simulink model "soru2"  (R2019b)
settings: Solver=VariableStepAuto  StartTime=0.0  StopTime=50  RelTol=1e-3
libraries: fuzblock x20
settings Model: Creator=Mustafa_Sezer  LastModifiedBy=Mustafa_Sezer
settings SolverCC: AlgebraicLoopSolver=LineSearch

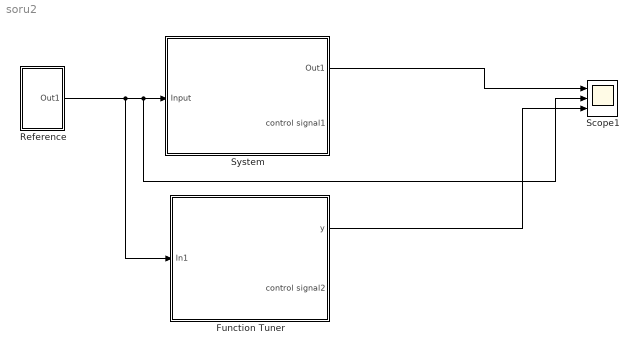
== system soru2 ==
  Function Tuner : Subsystem
  Reference : Subsystem
  Scope1 : Scope  NumInputPorts=3
  System : Subsystem
  wires:
  Function Tuner/1(y) -> Scope1/3
  Reference/1(Out1) -> Function Tuner/1(In1), Scope1/2, System/1(Input)
  System/1(Out1) -> Scope1/1

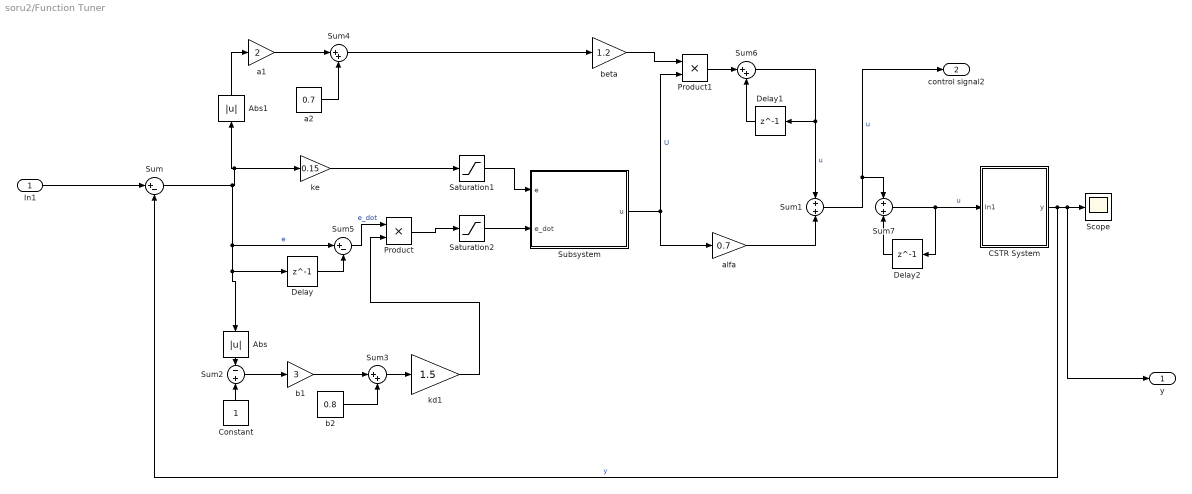
== system soru2/Function Tuner ==
  In1 : Inport
  Abs : Abs
  Abs1 : Abs
  CSTR System : Subsystem
  Constant : Constant  SampleTime=0.01
  Delay : Delay  DelayLength=1  SampleTime=0.1
  Delay1 : Delay  DelayLength=1  SampleTime=0.1
  Delay2 : Delay  DelayLength=1  SampleTime=0.1
  Product : Product
  Product1 : Product
  Saturation1 : Saturate  UpperLimit=1  LowerLimit=-1
  Saturation2 : Saturate  UpperLimit=1  LowerLimit=-1
  Scope : Scope
  Subsystem : Subsystem
  Sum : Sum  Inputs=|+-
  Sum1 : Sum
  Sum2 : Sum  Inputs=-+
  Sum3 : Sum  Inputs=|++
  Sum4 : Sum  Inputs=|++
  Sum5 : Sum  Inputs=|+-
  Sum6 : Sum  Inputs=|++
  Sum7 : Sum
  "a1 " : Gain  Gain=2
  a2 : Constant  Value=0.7  SampleTime=0.1
  "alfa " : Gain  Gain=0.7
  b1 : Gain  Gain=3
  b2 : Constant  Value=0.8  SampleTime=0.1
  beta : Gain  Gain=1.2
  kd1 : Gain  Gain=1.5
  ke : Gain  Gain=0.15
  y : Outport
  control signal2 : Outport  Port=2
  wires:
  "alfa "/1 -> Sum1/2
  ke/1 -> Saturation1/1
  Sum4/1 -> beta/1
  beta/1 -> Product1/1
  kd1/1 -> Product/2
  Product1/1 -> Sum6/1
  Sum3/1 -> kd1/1
  b1/1 -> Sum3/1
  Constant/1 -> Sum2/2
  Sum2/1 -> b1/1
  Abs/1 -> Sum2/1
  "a1 "/1 -> Sum4/1
  Subsystem/1(u) -> "alfa "/1, Product1/2  "U"
  Product/1 -> Saturation2/1
  Abs1/1 -> "a1 "/1
  CSTR System/1(y) -> y/1, Scope/1, Sum/2  "y"
  a2/1 -> Sum4/2
  Sum1/1 -> control signal2/1, Sum7/1  "u"
  b2/1 -> Sum3/2
  In1/1 -> Sum/1
  Saturation1/1 -> Subsystem/1(e)
  Saturation2/1 -> Subsystem/2(e_dot)
  Delay/1 -> Sum5/2
  Sum/1 -> Sum5/1, Abs/1, Delay/1, Abs1/1, ke/1  "e"
  Sum5/1 -> Product/1  "e_dot"
  Sum6/1 -> Delay1/1, Sum1/1  "u"
  Delay1/1 -> Sum6/2
  Delay2/1 -> Sum7/2
  Sum7/1 -> CSTR System/1(In1), Delay2/1  "u"

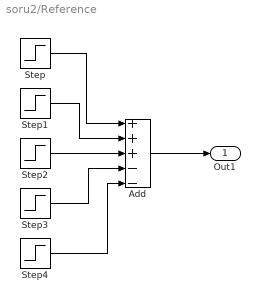
== system soru2/Reference ==
  Add : Sum  Inputs=+++--
  Step : Step  Time=0  After=0.4  SampleTime=0.1
  Step1 : Step  Time=10  After=0.1  SampleTime=0.1
  Step2 : Step  Time=20  After=0.1  SampleTime=0.1
  Step3 : Step  Time=30  After=0.1  SampleTime=0.1
  Step4 : Step  Time=40  After=0.1  SampleTime=0.1
  Out1 : Outport
  wires:
  Step1/1 -> Add/2
  Step/1 -> Add/1
  Add/1 -> Out1/1
  Step3/1 -> Add/4
  Step4/1 -> Add/5
  Step2/1 -> Add/3

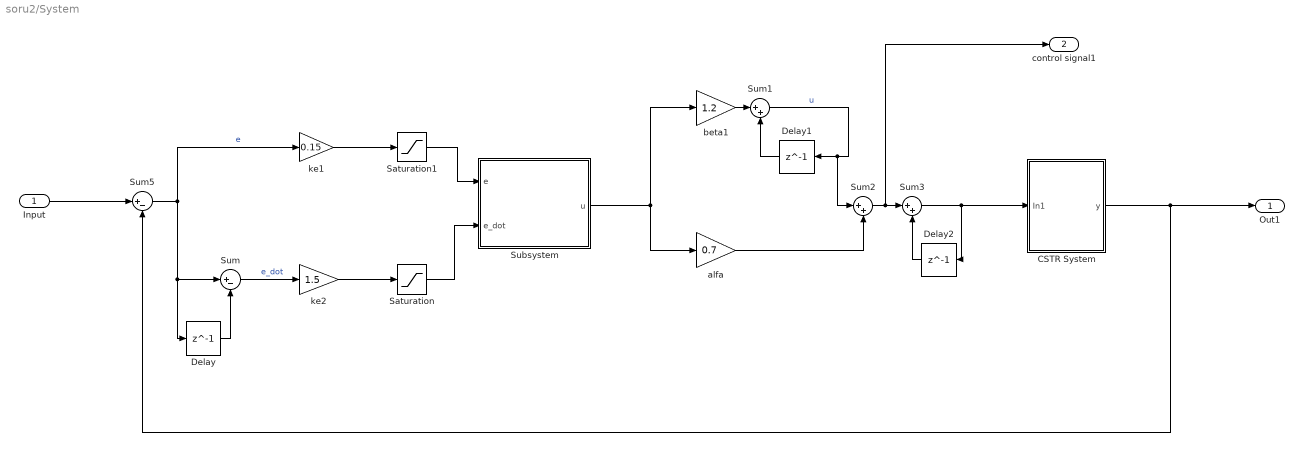
== system soru2/System ==
  Input : Inport
  CSTR System : Subsystem
  Delay : Delay  DelayLength=1  SampleTime=0.1
  Delay1 : Delay  DelayLength=1  SampleTime=0.1
  Delay2 : Delay  DelayLength=1  SampleTime=0.1
  Saturation : Saturate  UpperLimit=1  LowerLimit=-1
  Saturation1 : Saturate  UpperLimit=1  LowerLimit=-1
  Subsystem : Subsystem
  Sum : Sum  Inputs=|+-
  Sum1 : Sum  Inputs=|++
  Sum2 : Sum  Inputs=|++
  Sum3 : Sum  Inputs=|++
  Sum5 : Sum  Inputs=|+-
  alfa : Gain  Gain=0.7
  beta1 : Gain  Gain=1.2
  ke1 : Gain  Gain=0.15
  ke2 : Gain  Gain=1.5
  Out1 : Outport
  control signal1 : Outport  Port=2
  wires:
  beta1/1 -> Sum1/1
  Sum/1 -> ke2/1  "e_dot"
  Input/1 -> Sum5/1
  Sum5/1 -> Delay/1, Sum/1, ke1/1  "e"
  Sum1/1 -> Sum2/1, Delay1/1  "u"
  Subsystem/1(u) -> beta1/1, alfa/1
  ke1/1 -> Saturation1/1
  ke2/1 -> Saturation/1
  Delay/1 -> Sum/2
  Delay1/1 -> Sum1/2
  Saturation/1 -> Subsystem/2(e_dot)
  Sum2/1 -> control signal1/1, Sum3/1
  alfa/1 -> Sum2/2
  Saturation1/1 -> Subsystem/1(e)
  Sum3/1 -> Delay2/1, CSTR System/1(In1)
  Delay2/1 -> Sum3/2
  CSTR System/1(y) -> Sum5/2, Out1/1

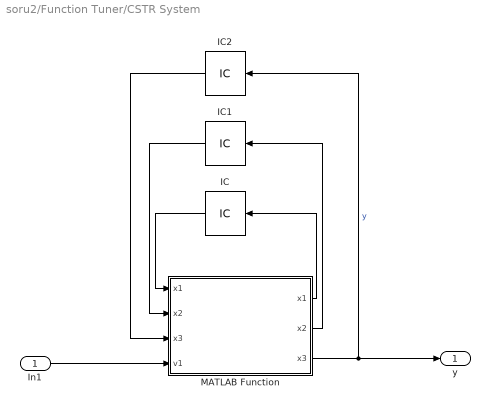
== system soru2/Function Tuner/CSTR System ==
  In1 : Inport
  IC : InitialCondition  Value=0.31
  IC1 : InitialCondition  Value=0.71
  IC2 : InitialCondition  Value=0.5
  MATLAB Function : MATLAB Function  TreatAsAtomicUnit=on
  y : Outport
  wires:
  IC1/1 -> MATLAB Function/2("x2 ")
  MATLAB Function/2(x2) -> IC1/1
  IC/1 -> MATLAB Function/1("x1 ")
  In1/1 -> MATLAB Function/4(v1)
  MATLAB Function/1(x1) -> IC/1
  IC2/1 -> MATLAB Function/3("x3 ")
  MATLAB Function/3(x3) -> y/1, IC2/1  "y"

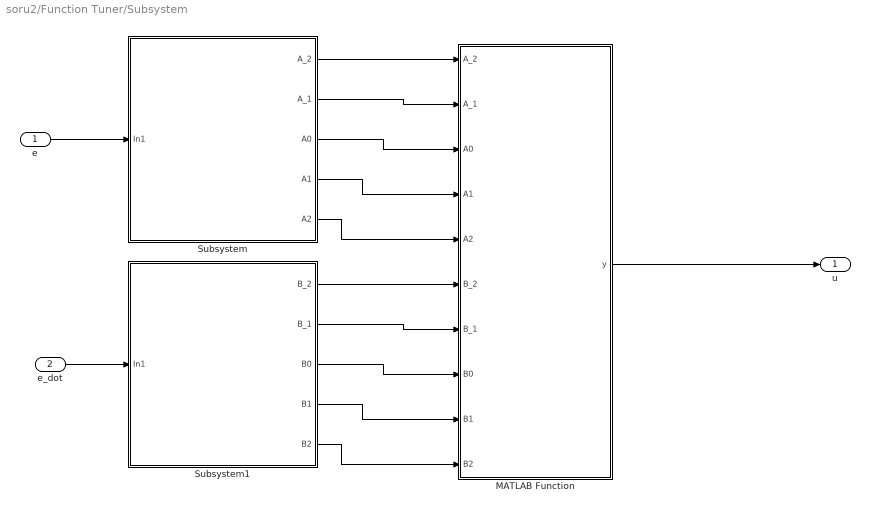
== system soru2/Function Tuner/Subsystem ==
  e : Inport
  e_dot : Inport  Port=2
  MATLAB Function : MATLAB Function  TreatAsAtomicUnit=on
  Subsystem : Subsystem
  Subsystem1 : Subsystem
  u : Outport
  wires:
  MATLAB Function/1(y) -> u/1
  Subsystem/5(A2) -> MATLAB Function/5(A2)
  Subsystem/4(A1) -> MATLAB Function/4(A1)
  Subsystem/3(A0) -> MATLAB Function/3(A0)
  Subsystem/2(A_1) -> MATLAB Function/2(A_1)
  Subsystem/1(A_2) -> MATLAB Function/1(A_2)
  Subsystem1/1(B_2) -> MATLAB Function/6(B_2)
  Subsystem1/2(B_1) -> MATLAB Function/7(B_1)
  Subsystem1/3(B0) -> MATLAB Function/8(B0)
  Subsystem1/4(B1) -> MATLAB Function/9(B1)
  Subsystem1/5(B2) -> MATLAB Function/10(B2)
  e/1 -> Subsystem/1(In1)
  e_dot/1 -> Subsystem1/1(In1)

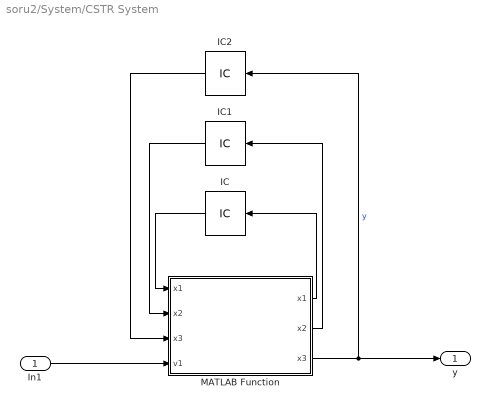
== system soru2/System/CSTR System ==
  In1 : Inport
  IC : InitialCondition  Value=0.31
  IC1 : InitialCondition  Value=0.71
  IC2 : InitialCondition  Value=0.5
  MATLAB Function : MATLAB Function  TreatAsAtomicUnit=on
  y : Outport
  wires:
  IC1/1 -> MATLAB Function/2("x2 ")
  MATLAB Function/2(x2) -> IC1/1
  IC/1 -> MATLAB Function/1("x1 ")
  In1/1 -> MATLAB Function/4(v1)
  MATLAB Function/1(x1) -> IC/1
  IC2/1 -> MATLAB Function/3("x3 ")
  MATLAB Function/3(x3) -> y/1, IC2/1  "y"

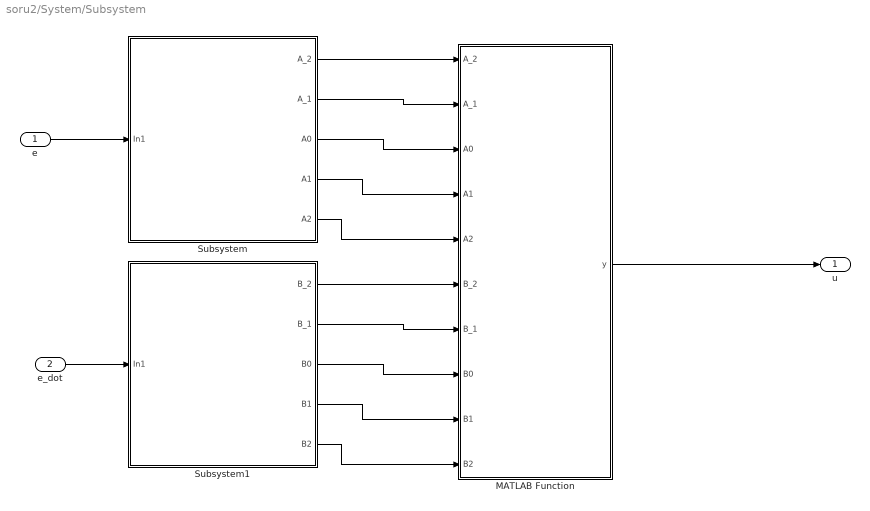
== system soru2/System/Subsystem ==
  e : Inport
  e_dot : Inport  Port=2
  MATLAB Function : MATLAB Function  TreatAsAtomicUnit=on
  Subsystem : Subsystem
  Subsystem1 : Subsystem
  u : Outport
  wires:
  MATLAB Function/1(y) -> u/1
  Subsystem/5(A2) -> MATLAB Function/5(A2)
  Subsystem/4(A1) -> MATLAB Function/4(A1)
  Subsystem/3(A0) -> MATLAB Function/3(A0)
  Subsystem/2(A_1) -> MATLAB Function/2(A_1)
  Subsystem/1(A_2) -> MATLAB Function/1(A_2)
  Subsystem1/1(B_2) -> MATLAB Function/6(B_2)
  Subsystem1/2(B_1) -> MATLAB Function/7(B_1)
  Subsystem1/3(B0) -> MATLAB Function/8(B0)
  Subsystem1/4(B1) -> MATLAB Function/9(B1)
  Subsystem1/5(B2) -> MATLAB Function/10(B2)
  e/1 -> Subsystem/1(In1)
  e_dot/1 -> Subsystem1/1(In1)

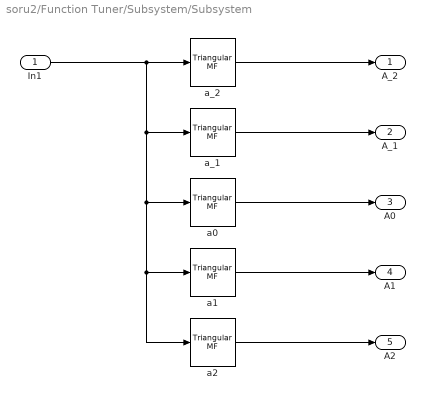
== system soru2/Function Tuner/Subsystem/Subsystem ==
  In1 : Inport
  a0 : fuzblock/Membership  Functions/Triangular MF  a=-0.4  b=0  c=0.4
      settings: SourceProductName=Fuzzy Logic Toolbox  SourceProductBaseCode=FL
  a1 : fuzblock/Membership  Functions/Triangular MF  a=0  b=0.4  c=1
      settings: SourceProductName=Fuzzy Logic Toolbox  SourceProductBaseCode=FL
  a2 : fuzblock/Membership  Functions/Triangular MF  a=0.4  b=1  c=1
      settings: SourceProductName=Fuzzy Logic Toolbox  SourceProductBaseCode=FL
  a_1 : fuzblock/Membership  Functions/Triangular MF  a=-1  b=-0.4  c=0
      settings: SourceProductName=Fuzzy Logic Toolbox  SourceProductBaseCode=FL
  a_2 : fuzblock/Membership  Functions/Triangular MF  a=-1  b=-1  c=-0.4
      settings: SourceProductName=Fuzzy Logic Toolbox  SourceProductBaseCode=FL
  A_2 : Outport
  A_1 : Outport  Port=2
  A0 : Outport  Port=3
  A1 : Outport  Port=4
  A2 : Outport  Port=5
  wires:
  a_2/1 -> A_2/1
  a1/1 -> A1/1
  a2/1 -> A2/1
  a_1/1 -> A_1/1
  a0/1 -> A0/1
  In1/1 -> a2/1, a1/1, a0/1, a_1/1, a_2/1

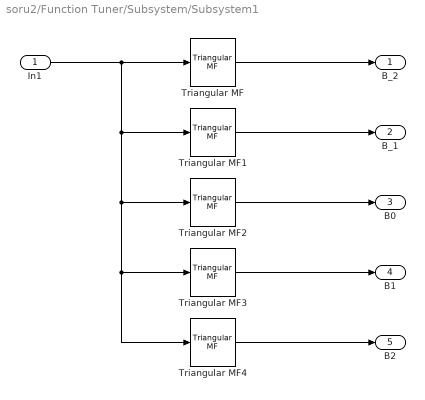
== system soru2/Function Tuner/Subsystem/Subsystem1 ==
  In1 : Inport
  Triangular MF : fuzblock/Membership  Functions/Triangular MF  a=-1  b=-1  c=-0.4
      settings: SourceProductName=Fuzzy Logic Toolbox  SourceProductBaseCode=FL
  Triangular MF1 : fuzblock/Membership  Functions/Triangular MF  a=-1  b=-0.4  c=0
      settings: SourceProductName=Fuzzy Logic Toolbox  SourceProductBaseCode=FL
  Triangular MF2 : fuzblock/Membership  Functions/Triangular MF  a=-0.4  b=0  c=0.4
      settings: SourceProductName=Fuzzy Logic Toolbox  SourceProductBaseCode=FL
  Triangular MF3 : fuzblock/Membership  Functions/Triangular MF  a=0  b=0.4  c=1
      settings: SourceProductName=Fuzzy Logic Toolbox  SourceProductBaseCode=FL
  Triangular MF4 : fuzblock/Membership  Functions/Triangular MF  a=0.4  b=1  c=1
      settings: SourceProductName=Fuzzy Logic Toolbox  SourceProductBaseCode=FL
  B_2 : Outport
  B_1 : Outport  Port=2
  B0 : Outport  Port=3
  B1 : Outport  Port=4
  B2 : Outport  Port=5
  wires:
  In1/1 -> Triangular MF4/1, Triangular MF3/1, Triangular MF2/1, Triangular MF1/1, Triangular MF/1
  Triangular MF/1 -> B_2/1
  Triangular MF4/1 -> B2/1
  Triangular MF2/1 -> B0/1
  Triangular MF1/1 -> B_1/1
  Triangular MF3/1 -> B1/1

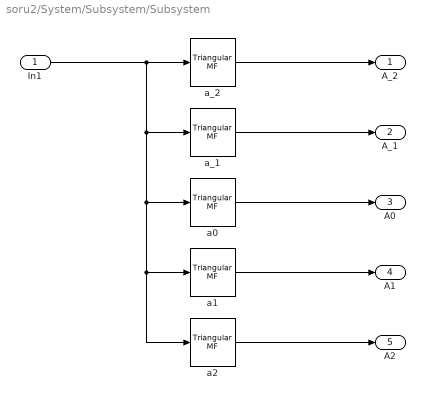
== system soru2/System/Subsystem/Subsystem ==
  In1 : Inport
  a0 : fuzblock/Membership  Functions/Triangular MF  a=-0.4  b=0  c=0.4
      settings: SourceProductName=Fuzzy Logic Toolbox  SourceProductBaseCode=FL
  a1 : fuzblock/Membership  Functions/Triangular MF  a=0  b=0.4  c=1
      settings: SourceProductName=Fuzzy Logic Toolbox  SourceProductBaseCode=FL
  a2 : fuzblock/Membership  Functions/Triangular MF  a=0.4  b=1  c=1
      settings: SourceProductName=Fuzzy Logic Toolbox  SourceProductBaseCode=FL
  a_1 : fuzblock/Membership  Functions/Triangular MF  a=-1  b=-0.4  c=0
      settings: SourceProductName=Fuzzy Logic Toolbox  SourceProductBaseCode=FL
  a_2 : fuzblock/Membership  Functions/Triangular MF  a=-1  b=-1  c=-0.4
      settings: SourceProductName=Fuzzy Logic Toolbox  SourceProductBaseCode=FL
  A_2 : Outport
  A_1 : Outport  Port=2
  A0 : Outport  Port=3
  A1 : Outport  Port=4
  A2 : Outport  Port=5
  wires:
  a_2/1 -> A_2/1
  a1/1 -> A1/1
  a2/1 -> A2/1
  a_1/1 -> A_1/1
  a0/1 -> A0/1
  In1/1 -> a2/1, a1/1, a0/1, a_1/1, a_2/1

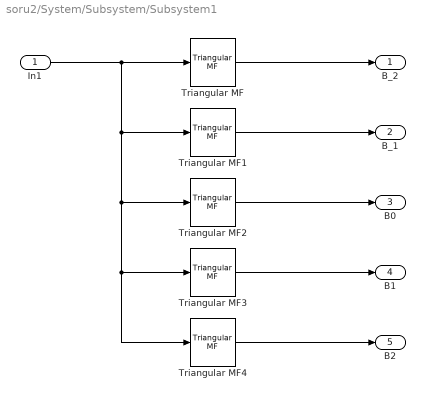
== system soru2/System/Subsystem/Subsystem1 ==
  In1 : Inport
  Triangular MF : fuzblock/Membership  Functions/Triangular MF  a=-1  b=-1  c=-0.4
      settings: SourceProductName=Fuzzy Logic Toolbox  SourceProductBaseCode=FL
  Triangular MF1 : fuzblock/Membership  Functions/Triangular MF  a=-1  b=-0.4  c=0
      settings: SourceProductName=Fuzzy Logic Toolbox  SourceProductBaseCode=FL
  Triangular MF2 : fuzblock/Membership  Functions/Triangular MF  a=-0.4  b=0  c=0.4
      settings: SourceProductName=Fuzzy Logic Toolbox  SourceProductBaseCode=FL
  Triangular MF3 : fuzblock/Membership  Functions/Triangular MF  a=0  b=0.4  c=1
      settings: SourceProductName=Fuzzy Logic Toolbox  SourceProductBaseCode=FL
  Triangular MF4 : fuzblock/Membership  Functions/Triangular MF  a=0.4  b=1  c=1
      settings: SourceProductName=Fuzzy Logic Toolbox  SourceProductBaseCode=FL
  B_2 : Outport
  B_1 : Outport  Port=2
  B0 : Outport  Port=3
  B1 : Outport  Port=4
  B2 : Outport  Port=5
  wires:
  In1/1 -> Triangular MF4/1, Triangular MF3/1, Triangular MF2/1, Triangular MF1/1, Triangular MF/1
  Triangular MF/1 -> B_2/1
  Triangular MF4/1 -> B2/1
  Triangular MF2/1 -> B0/1
  Triangular MF1/1 -> B_1/1
  Triangular MF3/1 -> B1/1

== matlab function soru2/System/Subsystem/MATLAB Function ==
  data: A_2 input; y output; A_1 input; A0 input; A1 input; A2 input; B_2 input; B_1 input; B0 input; B1 input; B2 input
function y = fcn(A_2, A_1, A0, A1, A2, B_2, B_1, B0, B1, B2)
u_2_2 = -1;
u_2_1 = -0.7;
u_20 = -0.5;
u_21 = -0.3;
u_22 = 0;

u_1_2 = -0.7;
u_1_1 = -0.4;
u_10 = -0.2;
u_11 = 0;
u_12 = 0.3;

u0_2 = -0.5;
u0_1 = -0.2;
u00 = 0;
u01 = 0.2;
u02 = 0.5;

u1_2 = -0.3;
u1_1 = 0;
u10 = 0.2;
u11 = 0.4;
u12 = 0.7;

u2_2 = 0;
u2_1 = 0.3;
u20 = 0.5;
u21 = 0.7;
u22 = 1;

if ((A0==0) && (A1==0) && (A2==0)) % A_1 ve A_2
    
    if((B0==0) && (B1==0) && (B2==0) && (B_1~= 0) && (B_2~= 0))
        y = A_2*B_2*u_2_2 + A_2*B_1*u_2_1 + A_1*B_1*u_1_1 + A_1*B_2*u_1_2;
    
    elseif((B_2==0) && (B1==0) && (B2==0) && (B_1~= 0) && (B0~= 0))
        y = A_2*B_1*u_2_1 + A_2*B0*u_20 + A_1*B_1*u_1_1 + A_1*B0*u_10;
    
    elseif((B_2==0) && (B_1==0) && (B2==0) && (B0~= 0) && (B1~= 0))
        y = A_2*B0*u_20 + A_2*B1*u_21 + A_1*B0*u_10 + A_1*B1*u_11;
    
    elseif((B0==0) && (B_1==0) && (B_2==0) && (B1~= 0) && (B2~= 0))
        y = A_2*B1*u_21 + A_2*B2*u_22 + A_1*B1*u_11 + A_1*B2*u_12;
    
    elseif((B_1==0) && (B0==0) && (B1==0) && (B2==0))
        y = A_2*B_2*u_2_2 + A_1*B_2*u_1_2;
    
    elseif((B_2==0) && (B0==0) && (B1==0) && (B2==0))
        y = A_2*B_1*u_2_1 + A_1*B_1*u_1_1;
    
    elseif((B_2==0) && (B_1==0) && (B1==0) && (B2==0))
        y = A_2*B0*u_20 + A_1*B0*u_10;
    
    elseif((B_2==0) && (B_1==0) && (B0==0) && (B2==0))
        y = A_2*B1*u_21 + A_1*B1*u_11;
    
    elseif((B_2==0) && (B_1==0) && (B0==0) && (B1==0))
        y = A_2*B2*u_22 + A_1*B2*u_12;
    
    else
        y=0.5;
    end
    
elseif ((A_2==0) && (A1==0) && (A2==0)) % A_1 ve A0
    
    if((B0==0) && (B1==0) && (B2==0) && (B_1~= 0) && (B_2~= 0))
        y = A0*B_2*u0_2 + A0*B_1*u0_1 + A_1*B_1*u_1_1 + A_1*B_2*u_1_2;
    
    elseif((B_2==0) && (B1==0) && (B2==0) && (B_1~= 0) && (B0~= 0))
        y = A0*B_1*u0_1 + A0*B0*u00 + A_1*B_1*u_1_1 + A_1*B0*u_10;
    
    elseif((B_2==0) && (B_1==0) && (B2==0) && (B0~= 0) && (B1~= 0))
        y = A0*B0*u00 + A0*B1*u01 + A_1*B0*u_10 + A_1*B1*u_11;
    
    elseif((B0==0) && (B_1==0) && (B_2==0) && (B1~= 0) && (B2~= 0))
        y = A0*B1*u01 + A0*B2*u02 + A_1*B1*u_11 + A_1*B2*u_12;
    
    elseif((B_1==0) && (B0==0) && (B1==0) && (B2==0))
        y = A0*B_2*u0_2 + A_1*B_2*u_1_2;
    
    elseif((B_2==0) && (B0==0) && (B1==0) && (B2==0))
        y = A0*B_1*u0_1 + A_1*B_1*u_1_1;
    
    elseif((B_2==0) && (B_1==0) && (B1==0) && (B2==0))
        y = A0*B0*u00 + A_1*B0*u_10;
    
    elseif((B_2==0) && (B_1==0) && (B0==0) && (B2==0))
        y = A0*B1*u01 + A_1*B1*u_11;
    
    elseif((B_2==0) && (B_1==0) && (B0==0) && (B1==0))
        y = A0*B2*u02 + A_1*B2*u_12;
    
    else
        y=0.5;
    end
    
elseif ((A_2==0) && (A_1==0) && (A2==0)) % A1 ve A0
    
    if((B0==0) && (B1==0) && (B2==0) && (B_1~= 0) && (B_2~= 0))
        y = A0*B_2*u0_2 + A0*B_1*u0_1 + A1*B_1*u1_1 + A1*B_2*u1_2;
    
    elseif((B_2==0) && (B1==0) && (B2==0) && (B_1~= 0) && (B0~= 0))
        y = A0*B_1*u0_1 + A0*B0*u00 + A1*B_1*u1_1 + A1*B0*u10;
    
    elseif((B_2==0) && (B_1==0) && (B2==0) && (B0~= 0) && (B1~= 0))
        y = A0*B0*u00 + A0*B1*u01 + A1*B0*u10 + A1*B1*u11;
    
    elseif((B0==0) && (B_1==0) && (B_2==0) && (B1~= 0) && (B2~= 0))
        y = A0*B1*u01 + A0*B2*u02 + A1*B1*u11 + A1*B2*u12;
    
    elseif((B_1==0) && (B0==0) && (B1==0) && (B2==0))
        y = A0*B_2*u0_2 + A1*B_2*u1_2;
    
    elseif((B_2==0) && (B0==0) && (B1==0) && (B2==0))
        y = A0*B_1*u0_1 + A1*B_1*u1_1;
    
    elseif((B_2==0) && (B_1==0) && (B1==0) && (B2==0))
        y = A0*B0*u00 + A1*B0*u10;
    
    elseif((B_2==0) && (B_1==0) && (B0==0) && (B2==0))
        y = A0*B1*u01 + A1*B1*u11;
    
    elseif((B_2==0) && (B_1==0) && (B0==0) && (B1==0))
        y = A0*B2*u02 + A1*B2*u12;
    
    else
        y=0.5;
    end
    
elseif ((A_2==0) && (A_1==0) && (A0==0)) % A1 ve A2
    
    if((B0==0) && (B1==0) && (B2==0) && (B_1~= 0) && (B_2~= 0))
        y = A2*B_2*u2_2 + A2*B_1*u2_1 + A1*B_1*u1_1 + A1*B_2*u1_2;
    
    elseif((B_2==0) && (B1==0) && (B2==0) && (B_1~= 0) && (B0~= 0))
        y = A2*B_1*u2_1 + A2*B0*u20 + A1*B_1*u1_1 + A1*B0*u10;
    
    elseif((B_2==0) && (B_1==0) && (B2==0) && (B0~= 0) && (B1~= 0))
        y = A2*B0*u20 + A2*B1*u21 + A1*B0*u10 + A1*B1*u11;
    
    elseif((B0==0) && (B_1==0) && (B_2==0) && (B1~= 0) && (B2~= 0))
        y = A2*B1*u21 + A2*B2*u22 + A1*B1*u11 + A1*B2*u12;
    
    elseif((B_1==0) && (B0==0) && (B1==0) && (B2==0))
        y = A2*B_2*u2_2 + A1*B_2*u1_2;
    
    elseif((B_2==0) && (B0==0) && (B1==0) && (B2==0))
        y = A2*B_1*u2_1 + A1*B_1*u1_1;
    
    elseif((B_2==0) && (B_1==0) && (B1==0) && (B2==0))
        y = A2*B0*u20 + A1*B0*u10;
    
    elseif((B_2==0) && (B_1==0) && (B0==0) && (B2==0))
        y = A2*B1*u21 + A1*B1*u11;
    
    elseif((B_2==0) && (B_1==0) && (B0==0) && (B1==0))
        y = A2*B2*u22 + A1*B2*u12;
    
    else
        y=0.5;
    end
else
    y=0.5;
end

== matlab function soru2/System/CSTR System/MATLAB Function ==
  data: x1 input; x1 output; x2 input; x3 input; v1 input; x2 output; x3 output
% Runge Kutta method for CSTR 
% Da1, Da2, Da3, d2 are CSTR parameters
% v1 is control input.
% h is the sampling time.
% x1, x2, x3 are the states of the system.

function  [x1,x2,x3]=CSTR_runga_kutta_new(x1,x2,x3,v1)
Da1 = 3; Da2 = 0.5; Da3 = 1; d2 = 1; h = 0.1;

k1x1=1-x1-Da1*x1+Da2*x2*x2;
k1x2=-x2+Da1*x1-Da2*x2*x2-Da3*d2*x2*x2+v1;
k1x3=-x3+Da3*d2*x2*x2;



k2x1=1-(x1+h*k1x1/2)-Da1*(x1+h*k1x1/2)+Da2*(x2+h*k1x2/2)*(x2+h*k1x2/2);
k2x2=-(x2+h*k1x2/2)+Da1*(x1+h*k1x1/2)-Da2*(x2+h*k1x2/2)*(x2+h*k1x2/2)-Da3*d2*(x2+h*k1x2/2)*(x2+h*k1x2/2)+v1;
k2x3=-(x3+h*k1x3/2 )+Da3*d2*(x2+h*k1x2/2)*(x2+h*k1x2/2);


k3x1=1-(x1+h*k2x1/2)-Da1*(x1+h*k2x1/2)+Da2*(x2+h*k2x2/2)*(x2+h*k2x2/2);
k3x2=-(x2+h*k2x2/2)+Da1*(x1+h*k2x1/2)-Da2*(x2+h*k2x2/2)*(x2+h*k2x2/2)-Da3*d2*(x2+h*k2x2/2)*(x2+h*k2x2/2)+v1;
k3x3=-(x3+h*k2x3/2)+Da3*d2*(x2+h*k2x2/2)*(x2+h*k2x2/2);



k4x1=1-(x1+h*k3x1)-Da1*(x1+h*k3x1)+Da2*(x2+h*k3x2)*(x2+h*k3x2);
k4x2=-(x2+h*k3x2)+Da1*(x1+h*k3x1)-Da2*(x2+h*k3x2)*(x2+h*k3x2)-Da3*d2*(x2+h*k3x2)*(x2+h*k3x2)+v1;
k4x3=-(x3+h*k3x3)+Da3*d2*(x2+h*k3x2)*(x2+h*k3x2);



x1=x1+(h/6)*(k1x1+2*k2x1+2*k3x1+k4x1);
x2=x2+(h/6)*(k1x2+2*k2x2+2*k3x2+k4x2);
x3=x3+(h/6)*(k1x3+2*k2x3+2*k3x3+k4x3);

== matlab function soru2/Function Tuner/Subsystem/MATLAB Function ==
  data: A_2 input; y output; A_1 input; A0 input; A1 input; A2 input; B_2 input; B_1 input; B0 input; B1 input; B2 input
function y = fcn(A_2, A_1, A0, A1, A2, B_2, B_1, B0, B1, B2)
u_2_2 = -1;
u_2_1 = -0.7;
u_20 = -0.5;
u_21 = -0.3;
u_22 = 0;

u_1_2 = -0.7;
u_1_1 = -0.4;
u_10 = -0.2;
u_11 = 0;
u_12 = 0.3;

u0_2 = -0.5;
u0_1 = -0.2;
u00 = 0;
u01 = 0.2;
u02 = 0.5;

u1_2 = -0.3;
u1_1 = 0;
u10 = 0.2;
u11 = 0.4;
u12 = 0.7;

u2_2 = 0;
u2_1 = 0.3;
u20 = 0.5;
u21 = 0.7;
u22 = 1;

if ((A0==0) && (A1==0) && (A2==0)) % A_1 ve A_2
    
    if((B0==0) && (B1==0) && (B2==0) && (B_1~= 0) && (B_2~= 0))
        y = A_2*B_2*u_2_2 + A_2*B_1*u_2_1 + A_1*B_1*u_1_1 + A_1*B_2*u_1_2;
    
    elseif((B_2==0) && (B1==0) && (B2==0) && (B_1~= 0) && (B0~= 0))
        y = A_2*B_1*u_2_1 + A_2*B0*u_20 + A_1*B_1*u_1_1 + A_1*B0*u_10;
    
    elseif((B_2==0) && (B_1==0) && (B2==0) && (B0~= 0) && (B1~= 0))
        y = A_2*B0*u_20 + A_2*B1*u_21 + A_1*B0*u_10 + A_1*B1*u_11;
    
    elseif((B0==0) && (B_1==0) && (B_2==0) && (B1~= 0) && (B2~= 0))
        y = A_2*B1*u_21 + A_2*B2*u_22 + A_1*B1*u_11 + A_1*B2*u_12;
    
    elseif((B_1==0) && (B0==0) && (B1==0) && (B2==0))
        y = A_2*B_2*u_2_2 + A_1*B_2*u_1_2;
    
    elseif((B_2==0) && (B0==0) && (B1==0) && (B2==0))
        y = A_2*B_1*u_2_1 + A_1*B_1*u_1_1;
    
    elseif((B_2==0) && (B_1==0) && (B1==0) && (B2==0))
        y = A_2*B0*u_20 + A_1*B0*u_10;
    
    elseif((B_2==0) && (B_1==0) && (B0==0) && (B2==0))
        y = A_2*B1*u_21 + A_1*B1*u_11;
    
    elseif((B_2==0) && (B_1==0) && (B0==0) && (B1==0))
        y = A_2*B2*u_22 + A_1*B2*u_12;
    
    else
        y=0.5;
    end
    
elseif ((A_2==0) && (A1==0) && (A2==0)) % A_1 ve A0
    
    if((B0==0) && (B1==0) && (B2==0) && (B_1~= 0) && (B_2~= 0))
        y = A0*B_2*u0_2 + A0*B_1*u0_1 + A_1*B_1*u_1_1 + A_1*B_2*u_1_2;
    
    elseif((B_2==0) && (B1==0) && (B2==0) && (B_1~= 0) && (B0~= 0))
        y = A0*B_1*u0_1 + A0*B0*u00 + A_1*B_1*u_1_1 + A_1*B0*u_10;
    
    elseif((B_2==0) && (B_1==0) && (B2==0) && (B0~= 0) && (B1~= 0))
        y = A0*B0*u00 + A0*B1*u01 + A_1*B0*u_10 + A_1*B1*u_11;
    
    elseif((B0==0) && (B_1==0) && (B_2==0) && (B1~= 0) && (B2~= 0))
        y = A0*B1*u01 + A0*B2*u02 + A_1*B1*u_11 + A_1*B2*u_12;
    
    elseif((B_1==0) && (B0==0) && (B1==0) && (B2==0))
        y = A0*B_2*u0_2 + A_1*B_2*u_1_2;
    
    elseif((B_2==0) && (B0==0) && (B1==0) && (B2==0))
        y = A0*B_1*u0_1 + A_1*B_1*u_1_1;
    
    elseif((B_2==0) && (B_1==0) && (B1==0) && (B2==0))
        y = A0*B0*u00 + A_1*B0*u_10;
    
    elseif((B_2==0) && (B_1==0) && (B0==0) && (B2==0))
        y = A0*B1*u01 + A_1*B1*u_11;
    
    elseif((B_2==0) && (B_1==0) && (B0==0) && (B1==0))
        y = A0*B2*u02 + A_1*B2*u_12;
    
    else
        y=0.5;
    end
    
elseif ((A_2==0) && (A_1==0) && (A2==0)) % A1 ve A0
    
    if((B0==0) && (B1==0) && (B2==0) && (B_1~= 0) && (B_2~= 0))
        y = A0*B_2*u0_2 + A0*B_1*u0_1 + A1*B_1*u1_1 + A1*B_2*u1_2;
    
    elseif((B_2==0) && (B1==0) && (B2==0) && (B_1~= 0) && (B0~= 0))
        y = A0*B_1*u0_1 + A0*B0*u00 + A1*B_1*u1_1 + A1*B0*u10;
    
    elseif((B_2==0) && (B_1==0) && (B2==0) && (B0~= 0) && (B1~= 0))
        y = A0*B0*u00 + A0*B1*u01 + A1*B0*u10 + A1*B1*u11;
    
    elseif((B0==0) && (B_1==0) && (B_2==0) && (B1~= 0) && (B2~= 0))
        y = A0*B1*u01 + A0*B2*u02 + A1*B1*u11 + A1*B2*u12;
    
    elseif((B_1==0) && (B0==0) && (B1==0) && (B2==0))
        y = A0*B_2*u0_2 + A1*B_2*u1_2;
    
    elseif((B_2==0) && (B0==0) && (B1==0) && (B2==0))
        y = A0*B_1*u0_1 + A1*B_1*u1_1;
    
    elseif((B_2==0) && (B_1==0) && (B1==0) && (B2==0))
        y = A0*B0*u00 + A1*B0*u10;
    
    elseif((B_2==0) && (B_1==0) && (B0==0) && (B2==0))
        y = A0*B1*u01 + A1*B1*u11;
    
    elseif((B_2==0) && (B_1==0) && (B0==0) && (B1==0))
        y = A0*B2*u02 + A1*B2*u12;
    
    else
        y=0.5;
    end
    
elseif ((A_2==0) && (A_1==0) && (A0==0)) % A1 ve A2
    
    if((B0==0) && (B1==0) && (B2==0) && (B_1~= 0) && (B_2~= 0))
        y = A2*B_2*u2_2 + A2*B_1*u2_1 + A1*B_1*u1_1 + A1*B_2*u1_2;
    
    elseif((B_2==0) && (B1==0) && (B2==0) && (B_1~= 0) && (B0~= 0))
        y = A2*B_1*u2_1 + A2*B0*u20 + A1*B_1*u1_1 + A1*B0*u10;
    
    elseif((B_2==0) && (B_1==0) && (B2==0) && (B0~= 0) && (B1~= 0))
        y = A2*B0*u20 + A2*B1*u21 + A1*B0*u10 + A1*B1*u11;
    
    elseif((B0==0) && (B_1==0) && (B_2==0) && (B1~= 0) && (B2~= 0))
        y = A2*B1*u21 + A2*B2*u22 + A1*B1*u11 + A1*B2*u12;
    
    elseif((B_1==0) && (B0==0) && (B1==0) && (B2==0))
        y = A2*B_2*u2_2 + A1*B_2*u1_2;
    
    elseif((B_2==0) && (B0==0) && (B1==0) && (B2==0))
        y = A2*B_1*u2_1 + A1*B_1*u1_1;
    
    elseif((B_2==0) && (B_1==0) && (B1==0) && (B2==0))
        y = A2*B0*u20 + A1*B0*u10;
    
    elseif((B_2==0) && (B_1==0) && (B0==0) && (B2==0))
        y = A2*B1*u21 + A1*B1*u11;
    
    elseif((B_2==0) && (B_1==0) && (B0==0) && (B1==0))
        y = A2*B2*u22 + A1*B2*u12;
    
    else
        y=0.5;
    end
else
    y=0.5;
end

== matlab function soru2/Function Tuner/CSTR System/MATLAB Function ==
  data: x1 input; x1 output; x2 input; x3 input; v1 input; x2 output; x3 output
% Runge Kutta method for CSTR 
% Da1, Da2, Da3, d2 are CSTR parameters
% v1 is control input.
% h is the sampling time.
% x1, x2, x3 are the states of the system.

function  [x1,x2,x3]=CSTR_runga_kutta_new(x1,x2,x3,v1)
Da1 = 3; Da2 = 0.5; Da3 = 1; d2 = 1; h = 0.1;

k1x1=1-x1-Da1*x1+Da2*x2*x2;
k1x2=-x2+Da1*x1-Da2*x2*x2-Da3*d2*x2*x2+v1;
k1x3=-x3+Da3*d2*x2*x2;



k2x1=1-(x1+h*k1x1/2)-Da1*(x1+h*k1x1/2)+Da2*(x2+h*k1x2/2)*(x2+h*k1x2/2);
k2x2=-(x2+h*k1x2/2)+Da1*(x1+h*k1x1/2)-Da2*(x2+h*k1x2/2)*(x2+h*k1x2/2)-Da3*d2*(x2+h*k1x2/2)*(x2+h*k1x2/2)+v1;
k2x3=-(x3+h*k1x3/2 )+Da3*d2*(x2+h*k1x2/2)*(x2+h*k1x2/2);


k3x1=1-(x1+h*k2x1/2)-Da1*(x1+h*k2x1/2)+Da2*(x2+h*k2x2/2)*(x2+h*k2x2/2);
k3x2=-(x2+h*k2x2/2)+Da1*(x1+h*k2x1/2)-Da2*(x2+h*k2x2/2)*(x2+h*k2x2/2)-Da3*d2*(x2+h*k2x2/2)*(x2+h*k2x2/2)+v1;
k3x3=-(x3+h*k2x3/2)+Da3*d2*(x2+h*k2x2/2)*(x2+h*k2x2/2);



k4x1=1-(x1+h*k3x1)-Da1*(x1+h*k3x1)+Da2*(x2+h*k3x2)*(x2+h*k3x2);
k4x2=-(x2+h*k3x2)+Da1*(x1+h*k3x1)-Da2*(x2+h*k3x2)*(x2+h*k3x2)-Da3*d2*(x2+h*k3x2)*(x2+h*k3x2)+v1;
k4x3=-(x3+h*k3x3)+Da3*d2*(x2+h*k3x2)*(x2+h*k3x2);



x1=x1+(h/6)*(k1x1+2*k2x1+2*k3x1+k4x1);
x2=x2+(h/6)*(k1x2+2*k2x2+2*k3x2+k4x2);
x3=x3+(h/6)*(k1x3+2*k2x3+2*k3x3+k4x3);
